simulink model "PIDlonhiet_roirac_PIDso"  (R2018b)
settings: Solver=ode3  StartTime=0.0  StopTime=4000  FixedStep=T  RelTol=1e-3  EnableMultiTasking=on
values from neighbouring files (symbols this model uses):
  K = 150    [PIDroirac.m]
  T = 1.5    [PIDroirac.m]
  T1 = 480    [PIDroirac.m]
  T2 = 1440    [PIDroirac.m]
libraries: simulink x1
settings Model: Creator=Admin  LastModifiedBy=Admin
settings SolverCC: MaxConsecutiveMinStep=T
settings DataIOCC: LimitDataPoints=on  SaveFormat=Array
settings OptimizationCC: LifeSpan=inf
settings DebuggingCC: SFUnexpectedBacktrackingDiag=warning  SFNoUnconditionalDefaultTransitionDiag=warning  SFExecutionAtInitializationDiag=none
settings HardwareCC: ProdBitPerPointer=32  ProdBitPerSizeT=32  ProdBitPerPtrDiffT=32  ProdLargestAtomicFloat=None  ProdIntDivRoundTo=Undefined  ProdEndianess=Unspecified  ProdWordSize=32  ProdHWDeviceType=32-bit Generic
settings ModelReferenceCC: PropagateSignalLabelsOutOfModel=off
settings SFSimCC: SimUseLocalCustomCode=off
settings RTWCC: RTWUseLocalCustomCode=off
settings CodeAppCC: StateflowObjectComments=on
settings GRTTargetCC: TargetLangStandard=C89/C90 (ANSI)  GeneratePreprocessorConditionals=Disable all
settings ConfigComp: CovMetricSettings=dw  CovHtmlReporting=on  CovSaveCumulativeToWorkspaceVar=on  CovSaveSingleToWorkspaceVar=on  CovExternalEMLEnable=off

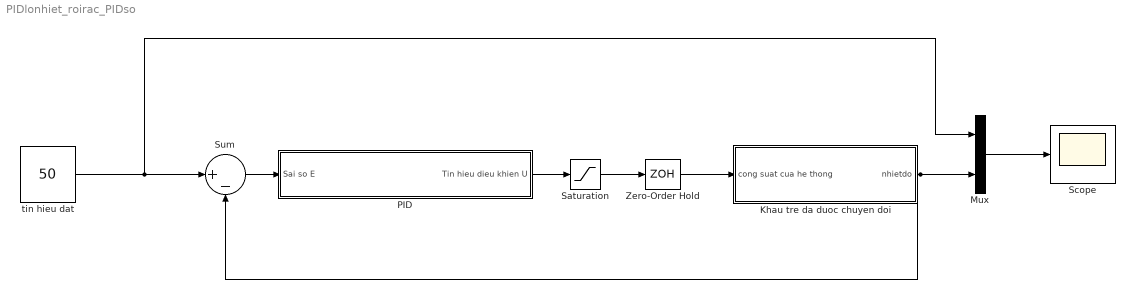
== system PIDlonhiet_roirac_PIDso ==
  "Khau tre da duoc chuyen doi " : Subsystem
  Mux : Mux  Inputs=2
  PID : Subsystem
  Saturation : Saturate  UpperLimit=1  LowerLimit=0
  Scope : Scope
  Sum : Sum  Inputs=|+-
  Zero-Order Hold : ZeroOrderHold  SampleTime=T
  tin hieu dat : Constant  Value=50
  wires:
  Mux/1 -> Scope/1
  Sum/1 -> PID/1(Sai so E)
  "Khau tre da duoc chuyen doi "/1(nhietdo) -> Sum/2, Mux/2
  tin hieu dat/1 -> Mux/1, Sum/1
  PID/1(Tin hieu dieu khien U) -> Saturation/1
  Saturation/1 -> Zero-Order Hold/1
  Zero-Order Hold/1 -> "Khau tre da duoc chuyen doi "/1(cong suat cua he thong)

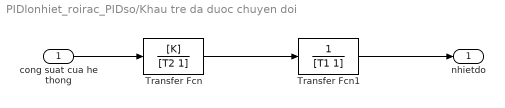
== system PIDlonhiet_roirac_PIDso/Khau tre da duoc chuyen doi  ==
  cong suat cua he thong : Inport
  Transfer Fcn : TransferFcn  Numerator=[K]  Denominator=[T2 1]
  Transfer Fcn1 : TransferFcn  Denominator=[T1 1]
  nhietdo : Outport
  wires:
  cong suat cua he thong/1 -> Transfer Fcn/1
  Transfer Fcn/1 -> Transfer Fcn1/1
  Transfer Fcn1/1 -> nhietdo/1

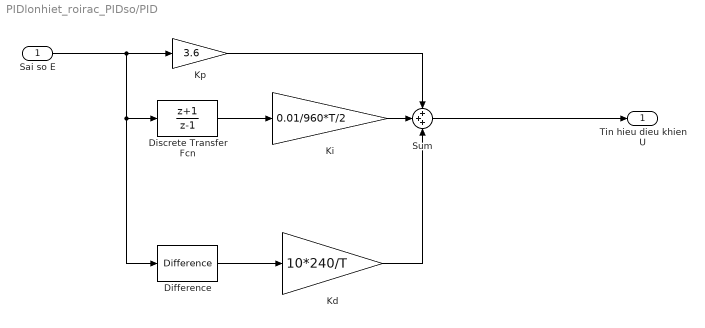
== system PIDlonhiet_roirac_PIDso/PID ==
  Sai so E : Inport
  Difference : simulink/Discrete/Difference  ICPrevInput=0.0  OutMin=[]  OutMax=[]  OutDataType=fixdt(1, 16)  OutScaling=2^-10  DoSatur=off
  Discrete Transfer Fcn : DiscreteTransferFcn  Numerator=[1 1]  Denominator=[1 -1]  SampleTime=T
  Kd : Gain  Gain=10*240/T
  Ki : Gain  Gain=0.01/960*T/2
  Kp : Gain  Gain=3.6
  Sum : Sum  Inputs=+++
  Tin hieu dieu khien U : Outport
  wires:
  Sai so E/1 -> Difference/1, Discrete Transfer Fcn/1, Kp/1
  Discrete Transfer Fcn/1 -> Ki/1
  Difference/1 -> Kd/1
  Kp/1 -> Sum/1
  Ki/1 -> Sum/2
  Kd/1 -> Sum/3
  Sum/1 -> Tin hieu dieu khien U/1
